simulink model "Udan_SOC"  (R2017b)
settings: Solver=FixedStepAuto  StartTime=0.0  StopTime=1000  FixedStep=0.1  RelTol=1e-3
values from neighbouring files (symbols this model uses):
  DenominatorOfIntegratorFactor = 100.0    [SOC_Stateflow.sldd]
  SOC_CalcSohLKT = 1.0    [SOC_Stateflow.sldd]
  SOC_CalcSOHTempLimit = 70.0    [SOC_Stateflow.sldd]
  SOC_CapPerCycle = 100.0    [SOC_Stateflow.sldd]
  SOC_CapTemp_HLimit = 200.0    [SOC_Stateflow.sldd]
  SOC_CapTemp_LLimit = 0.0    [SOC_Stateflow.sldd]
  Soc_ConfigInfo = 0    [SOC_Stateflow.sldd]
  SOC_DchgEndCalib = 0.0    [SOC_Stateflow.sldd]
  SOC_DiffVoltMin = 10.0    [SOC_Stateflow.sldd]
  SOC_DSOCJumpMax = 500.0    [SOC_Stateflow.sldd]
  SOC_EfficientHighLimit = 250.0    [SOC_Stateflow.sldd]
  SOC_EfficientLowLimit = 40.0    [SOC_Stateflow.sldd]
  SOC_EmptyAus = 0.0    [SOC_Stateflow.sldd]
  SOC_EnableOcv = 1.0    [SOC_Stateflow.sldd]
  SOC_END_CALIB_STATE : value not decoded    [SOC_Stateflow.sldd]
  SOC_HighRealSoc = 95.0    [SOC_Stateflow.sldd]
  SOC_LKTSohCycles = 0.0 1.0 10.0 20.0 30.0 40.0 50.0 60.0 70.0 80.0 90.0 100.0 110.0 120.0 130.0 140.0 150.0 160.0 170.0 180.0 190.0 200.0 210.0 220.0 230.0 240.0 250.0 260.0 270.0 280.0 290.0 300.0 310.0 320.0 330.0 340.0 350.0 360.0 370.0 380.0 390.0 400.0 410.0 420.0 430.0 440.0 450.0 460.0 470.0 480.0 490.0 500.0 510.0 520.0 530.0 540.0 550.0 560.0 570.0 580.0 590.0 600.0 610.0 620.0 630.0 640.0 650.0 660.0 670.0    [SOC_Stateflow.sldd]
  SOC_LKTSohTable = 1000.0 991.0 989.0 992.0 993.0 995.0 994.0 993.0 1000.0 997.0 1002.0 1000.0 992.0 1000.0 989.0 992.0 989.0 994.0 989.0 993.0 994.0 994.0 994.0 993.0 991.0 991.0 992.0 993.0 991.0 985.0 985.0 985.0 979.0 975.0 978.0 984.0 982.0 974.0 975.0 972.0 972.0 975.0 977.0 977.0 974.0 971.0 973.0 971.0 966.0 968.0 965.0 959.0 957.0 956.0 957.0 954.0 955.0 951.0 954.0 951.0 942.0 942.0 940.0 942.0 947.0 949.0    [SOC_Stateflow.sldd]
  SOC_LowRealSoc = 5.0    [SOC_Stateflow.sldd]
  SOC_NominalCap_AmS = 576000000.0    [SOC_Stateflow.sldd]
  SOC_NominalVol = 4000.0    [SOC_Stateflow.sldd]
  SOC_OCVTemp_HLimit = 106.0    [SOC_Stateflow.sldd]
  SOC_OCVTemp_LLimit = 29.0    [SOC_Stateflow.sldd]
  SOC_ShortCalibDSoc = 1.0    [SOC_Stateflow.sldd]
  SOC_SOCResolution = 10000.0    [SOC_Stateflow.sldd]
  SOC_SohCalcCapPercent = 8.0    [SOC_Stateflow.sldd]
  SOC_SohCalcHighLimit = 60.0    [SOC_Stateflow.sldd]
  SOC_SohCalcLowLimit = 10.0    [SOC_Stateflow.sldd]
  SOC_SohCalcMidLimit = 30.0    [SOC_Stateflow.sldd]
  SOC_SOHResolution = 1000.0    [SOC_Stateflow.sldd]
  SOC_State = <binary blob, 1163 chars, not shown>    [SOC_Stateflow.sldd]
  SOC_TempCap_CapBuffer : value not decoded    [SOC_Stateflow.sldd]
  SOC_TempCap_TempBuffer : value not decoded    [SOC_Stateflow.sldd]
  SocOcvCalib_ConfigInfo = 0.0    [SOC_Stateflow.sldd]
  SocOcvCalib_SocBuffer1 : value not decoded    [SOC_Stateflow.sldd]
  SocOcvCalib_TempBuffer : value not decoded    [SOC_Stateflow.sldd]
  SocOcvCalib_VoltageBuffer1 = 3300.0 3303.0 3305.0 3307.0 3310.0 3311.0 3313.0 3314.0 3316.0 3317.0 3319.0 3320.0 3322.0 3323.0 3325.0 3322.0 3323.0 3325.0 3310.0 3313.0 3315.0 3317.0 3320.0 3321.0 3323.0 3324.0 3326.0 3327.0 3329.0 3330.0 3332.0 3333.0 3335.0 3332.0 3333.0 3335.0 3320.0 3323.0 3325.0 3327.0 3330.0 3331.0 3333.0 3334.0 3336.0 3337.0 3339.0 3340.0 3342.0 3343.0 3345.0 3342.0 3343.0 3345.0 3330.0 3333.0 3335.0 3    [SOC_Stateflow.sldd]
  SOHCalibCycle = 10.0    [SOC_Stateflow.sldd]
undefined symbols (not defined in the file or in its folder): DatetimeM_GetReturnType, ParameterM_EeepParaIndexType, Soc_CumuLativeTypeType, SOC_EgthTempChgValue, Soc_EnergyBuffer, SOC_FithTempChgValue, SOC_FstSlowTempChgValue, SOC_FstTempChgValue, SOC_FthTempChgValue, SOC_MaxCap_AmS, SOC_SethTempChgValue, SOC_SixTempChgValue, SOC_SndSlowTempChgValue, SOC_SndTempChgValue, SOC_TrdSlowTempChgValue, SOC_TrdTempChgValue, SocDiagCalib_NoCalibReasonType
libraries: simulink x138, hdlsllib x24, dspindex x4
(part 4 of 10)

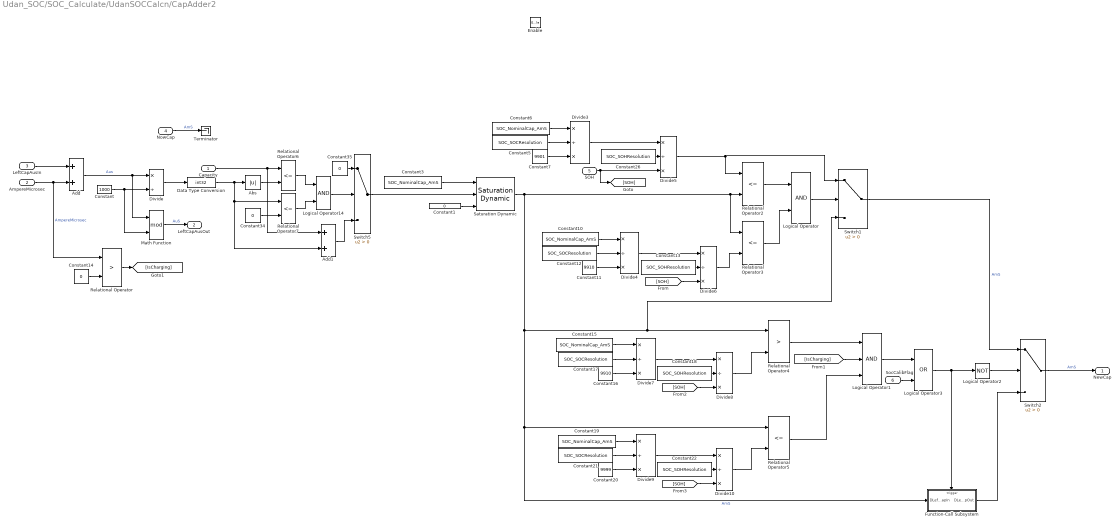
== system Udan_SOC/SOC_Calculate/UdanSOCCalcn/CapAdder2 ==
  Capacity : Inport
  AmpereMicrosec : Inport  Port=2
  LeftCapAusIn : Inport  Port=3
  NowCap : Inport  Port=4
  SOH : Inport  Port=5
  SocCalibFlag : Inport  Port=6  OutDataTypeStr=uint8  PortDimensions=[1]
  Enable : EnablePort
  Abs : Abs
  Add : Sum  AccumDataTypeStr=int32  OutDataTypeStr=int32
  Add1 : Sum  AccumDataTypeStr=uint32  OutDataTypeStr=uint32
  Constant : Constant  Value=1000  OutDataTypeStr=int32
  Constant1 : Constant  Value=0  OutDataTypeStr=uint32
  Constant{3,6,10,15,19} (5 alike) : Constant  Value=SOC_NominalCap_AmS
  Constant11 : Constant  Value=9910  OutDataTypeStr=uint16
  Constant{5,12,17,21} (4 alike) : Constant  Value=SOC_SOCResolution  OutDataTypeStr=uint16
  Constant{13,18,22,26} (4 alike) : Constant  Value=SOC_SOHResolution  OutDataTypeStr=uint16
  Constant14 : Constant  Value=0  OutDataTypeStr=uint8
  Constant16 : Constant  Value=9910  OutDataTypeStr=uint16
  Constant20 : Constant  Value=9999  OutDataTypeStr=uint16
  Constant34 : Constant  Value=0  OutDataTypeStr=uint8
  Constant35 : Constant  Value=0  OutDataTypeStr=uint8
  Constant7 : Constant  Value=9901  OutDataTypeStr=uint16
  Data Type Conversion : DataTypeConversion  OutDataTypeStr=int32
  Divide : Product  Inputs=*/  OutDataTypeStr=int32
  Divide{3..10} (8 alike) : Product  Inputs=*/*  OutDataTypeStr=uint32
  Function-Call Subsystem : Subsystem  TreatAsAtomicUnit=on
  Logical Operator : Logic  AllPortsSameDT=off  OutDataTypeStr=boolean
  Logical Operator1 : Logic  Inputs=3  AllPortsSameDT=off  OutDataTypeStr=boolean
  Logical Operator14 : Logic  AllPortsSameDT=off  OutDataTypeStr=boolean
  Logical Operator2 : Logic  Operator=NOT  AllPortsSameDT=off  OutDataTypeStr=boolean
  Logical Operator3 : Logic  Operator=OR  AllPortsSameDT=off  OutDataTypeStr=boolean
  Math Function : Math  Operator=mod  SaturateOnIntegerOverflow=on
  Relational Operator : RelationalOperator  Operator=>  OutDataTypeStr=boolean  RndMeth=Simplest
  Relational Operator{2..3,5..7} (5 alike) : RelationalOperator  Operator=<=  OutDataTypeStr=boolean  RndMeth=Simplest
  Relational Operator4 : RelationalOperator  Operator=>  OutDataTypeStr=boolean  RndMeth=Simplest
  Saturation Dynamic : simulink/Discontinuities/Saturation Dynamic  OutMin=[]  OutMax=[]  OutDataTypeStr=uint32  OutputDataTypeScalingMode=uint32  OutDataType=fixdt(1, 16)  OutScaling=2^-10  DoSatur=on
  Switch1 : Switch  Criteria=u2 > Threshold
  Switch2 : Switch  Criteria=u2 > Threshold
  Switch5 : Switch  Criteria=u2 > Threshold  OutDataTypeStr=uint32
  Terminator : Terminator
  NewCap : Outport
  LeftCapAusOut : Outport  Port=2
  wires:
  Add/1 -> Divide/1, Math Function/1  "Aus"
  Switch2/1 -> NewCap/1  "AmS"
  AmpereMicrosec/1 -> Relational Operator/1, Add/2  "AmpereMicrosec"
  Constant3/1 -> Saturation Dynamic/1
  Math Function/1 -> LeftCapAusOut/1  "AuS"
  Divide/1 -> Data Type Conversion/1
  Constant/1 -> Divide/2, Math Function/2
  LeftCapAusIn/1 -> Add/1
  Constant1/1 -> Saturation Dynamic/3
  Switch5/1 -> Saturation Dynamic/2
  Constant11/1 -> Divide4/3
  Relational Operator3/1 -> Logical Operator/2
  Divide6/1 -> Relational Operator3/2
  Logical Operator/1 -> Switch1/2
  Constant12/1 -> Divide4/2
  Constant5/1 -> Divide3/2
  Constant7/1 -> Divide3/3
  Relational Operator2/1 -> Logical Operator/1
  Saturation Dynamic/1 -> Relational Operator5/1, Function-Call Subsystem/1(DLeftCapIn), Switch1/3, Relational Operator4/1, Relational Operator3/1, Relational Operator2/2  "AmS"
  Divide5/1 -> Switch1/1, Relational Operator2/1
  Constant26/1 -> Divide5/2
  SOH/1 -> [SOH], Divide5/3
  Divide3/1 -> Divide5/1
  Constant13/1 -> Divide6/2
  Divide4/1 -> Divide6/1
  [SOH] -> Divide6/3
  Constant14/1 -> Relational Operator/2
  Relational Operator/1 -> [IsCharging]
  Divide7/1 -> Divide8/1
  Constant16/1 -> Divide7/3
  [SOH] -> Divide8/3
  Constant17/1 -> Divide7/2
  Constant18/1 -> Divide8/2
  Divide8/1 -> Relational Operator4/2
  Relational Operator4/1 -> Logical Operator1/1
  [IsCharging] -> Logical Operator1/2
  Logical Operator3/1 -> Logical Operator2/1, Function-Call Subsystem/Trigger
  Logical Operator2/1 -> Switch2/2
  Switch1/1 -> Switch2/1  "AmS"
  Function-Call Subsystem/1(DLeftCapOut) -> Switch2/3
  SocCalibFlag/1 -> Logical Operator3/2
  Logical Operator1/1 -> Logical Operator3/1
  Constant21/1 -> Divide9/2
  Divide10/1 -> Relational Operator5/2
  Constant20/1 -> Divide9/3
  [SOH] -> Divide10/3
  Constant22/1 -> Divide10/2
  Divide9/1 -> Divide10/1
  Relational Operator5/1 -> Logical Operator1/3
  Constant6/1 -> Divide3/1
  Constant10/1 -> Divide4/1
  Constant15/1 -> Divide7/1
  Constant19/1 -> Divide9/1
  NowCap/1 -> Terminator/1  "AmS"
  Logical Operator14/1 -> Switch5/2
  Relational Operator7/1 -> Logical Operator14/2
  Relational Operator6/1 -> Logical Operator14/1
  Constant35/1 -> Switch5/1
  Add1/1 -> Switch5/3
  Abs/1 -> Relational Operator6/2
  Capacity/1 -> Add1/1, Relational Operator6/1
  Constant34/1 -> Relational Operator7/2
  Data Type Conversion/1 -> Abs/1, Relational Operator7/1, Add1/2

== system Udan_SOC/SOC_Calculate/UdanSOCCalcn/ClearLeftCapWOCalib ==
  Trigger : TriggerPort  TriggerType=either  VariantControl=Variant  PortDimensions=1
  Constant2 : Constant  Value=0  OutDataTypeStr=uint32
  DchgPower2 : simulink/Sources/Enumerated Constant  OutDataTypeStr=Enum: ParameterM_EeepParaIndexType  Value=ParameterM_EeepParaIndexType.PARAMETERM_EEEP_LEFTCAP_WOCALIB_H_INDEX  SampleTime=inf
      settings: SourceProductName=Simulink
  DchgPower4 : simulink/Sources/Enumerated Constant  OutDataTypeStr=Enum: ParameterM_EeepParaIndexType  Value=ParameterM_EeepParaIndexType.PARAMETERM_EEEP_LEFTCAP_WOCALIB_L_INDEX  SampleTime=inf
      settings: SourceProductName=Simulink
  Subsystem : Subsystem  mask(EeepWrite_uint32){}
      mask help: EeepWrite_uint32
  wires:
  Constant2/1 -> Subsystem/1(data)
  DchgPower4/1 -> Subsystem/3(LowIndex)
  DchgPower2/1 -> Subsystem/2(HighIndex)

== system Udan_SOC/SOC_Calculate/UdanSOCCalcn/ClearLeftCapWOCalib2 ==
  Enable : EnablePort
  Constant : Constant  OutDataTypeStr=boolean
  Constant2 : Constant  Value=0  OutDataTypeStr=uint32
  Data Store Write : DataStoreWrite  DataStoreName=ChgClearWOCalibFlag
  DchgPower2 : simulink/Sources/Enumerated Constant  OutDataTypeStr=Enum: ParameterM_EeepParaIndexType  Value=ParameterM_EeepParaIndexType.PARAMETERM_EEEP_LEFTCAP_WOCALIB_H_INDEX  SampleTime=inf
      settings: SourceProductName=Simulink
  DchgPower4 : simulink/Sources/Enumerated Constant  OutDataTypeStr=Enum: ParameterM_EeepParaIndexType  Value=ParameterM_EeepParaIndexType.PARAMETERM_EEEP_LEFTCAP_WOCALIB_L_INDEX  SampleTime=inf
      settings: SourceProductName=Simulink
  Subsystem : Subsystem  mask(EeepWrite_uint32){}
      mask help: EeepWrite_uint32
  wires:
  DchgPower2/1 -> Subsystem/2(HighIndex)
  Constant2/1 -> Subsystem/1(data)
  DchgPower4/1 -> Subsystem/3(LowIndex)
  Constant/1 -> Data Store Write/1

== system Udan_SOC/SOC_Calculate/UdanSOCCalcn/ClearSOHCalcFlag ==
  Enable : EnablePort
  Constant1 : Constant  Value=65535  OutDataTypeStr=uint16
  DchgPower1 : simulink/Sources/Enumerated Constant  OutDataTypeStr=Enum: ParameterM_EeepParaIndexType  Value=ParameterM_EeepParaIndexType.PARAMETERM_EEEP_SOH_Full_INDEX  SampleTime=inf
      settings: SourceProductName=Simulink
  S-Function1 : S-Function  FunctionName=sfn_NVMWrite  SFunctionDeploymentMode=off  EnableBusSupport=off
  Terminator : Terminator
  wires:
  DchgPower1/1 -> S-Function1/1
  S-Function1/1 -> Terminator/1
  Constant1/1 -> S-Function1/2

== system Udan_SOC/SOC_Calculate/UdanSOCCalcn/Enabled Subsystem ==
  RtcTimeIn : Inport
  Enable : EnablePort
  Constant : Constant  OutDataTypeStr=boolean
  Data Store Write : DataStoreWrite  DataStoreName=LargeCurrentFlag
  RtcTimeOut : Outport
  wires:
  RtcTimeIn/1 -> RtcTimeOut/1
  Constant/1 -> Data Store Write/1

== system Udan_SOC/SOC_Calculate/UdanSOCCalcn/Function-Call Subsystem ==
  function : TriggerPort  TriggerType=falling  VariantControl=Variant
  Constant : Constant  Commented=on  Value=0  OutDataTypeStr=boolean
  Constant1 : Constant  Value=0  OutDataTypeStr=boolean
  Constant2 : Constant  Value=0  OutDataTypeStr=uint32
  Data Store Write : DataStoreWrite  Commented=on  DataStoreName=FullFnshFlag
  Data Store Write1 : DataStoreWrite  DataStoreName=ChgClearWOCalibFlag
  DchgPower2 : simulink/Sources/Enumerated Constant  OutDataTypeStr=Enum: ParameterM_EeepParaIndexType  Value=ParameterM_EeepParaIndexType.PARAMETERM_EEEP_LEFTCAP_WOCALIB_H_INDEX  SampleTime=inf
      settings: SourceProductName=Simulink
  DchgPower4 : simulink/Sources/Enumerated Constant  OutDataTypeStr=Enum: ParameterM_EeepParaIndexType  Value=ParameterM_EeepParaIndexType.PARAMETERM_EEEP_LEFTCAP_WOCALIB_L_INDEX  SampleTime=inf
      settings: SourceProductName=Simulink
  Subsystem : Subsystem  mask(EeepWrite_uint32){}
      mask help: EeepWrite_uint32
  wires:
  Constant/1 -> Data Store Write/1
  DchgPower4/1 -> Subsystem/3(LowIndex)
  Constant2/1 -> Subsystem/1(data)
  DchgPower2/1 -> Subsystem/2(HighIndex)
  Constant1/1 -> Data Store Write1/1

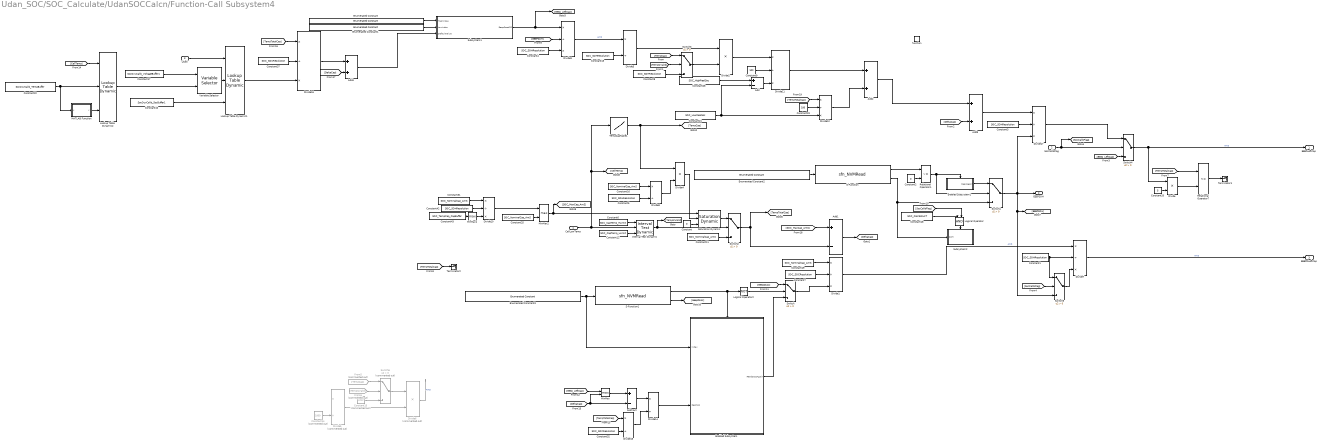
== system Udan_SOC/SOC_Calculate/UdanSOCCalcn/Function-Call Subsystem4 ==
  CellLowTemp : Inport
  SocCalibFlag : Inport  Port=2  OutDataTypeStr=uint8  PortDimensions=[1]
  UCell : Inport  Port=3
  function : TriggerPort  TriggerType=function-call  VariantControl=Variant
  Add : Sum  Inputs=+-  AccumDataTypeStr=uint8  OutDataTypeStr=uint8
  Add1 : Sum  Inputs=+-  OutDataTypeStr=int32
  Add2 : Sum  OutDataTypeStr=uint32
  Add3 : Sum  OutDataTypeStr=uint32
  Add4 : Sum
  Constant : Constant  Value=0  OutDataTypeStr=uint8
  Constant{1,3..5,8,13,42} (7 alike) : Constant  Value=SOC_SOHResolution  OutDataTypeStr=uint16
  Constant10 : Constant  Value=SocOcvCalib_SocBuffer1
  Constant{11,16,19,25,31} (5 alike) : Constant  Value=SOC_NominalCap_AmS
  Constant12 : Constant  Value=SOC_CapTemp_LLimit  OutDataTypeStr=uint8
  Constant14 : Constant  Commented=on  Value=1000  OutDataTypeStr=uint16
  Constant15 : Constant  Commented=on  Value=1000  OutDataTypeStr=uint16
  Constant17 : Constant  Value=SocOcvCalib_VoltageBuffer1
  Constant18 : Constant  Value=SOC_CalcSohLKT
  Constant2 : Constant  Value=0  OutDataTypeStr=uint8
  Constant20 : Constant  Value=5  OutDataTypeStr=uint8
  Constant21 : Constant  Value=SOC_LowRealSoc
  Constant22 : Constant  Value=SocOcvCalib_TempBuffer  OutDataTypeStr=uint8
  Constant23 : Constant  Value=100  OutDataTypeStr=uint8
  Constant28 : Constant  Value=SOC_HighRealSoc
  Constant32 : Constant  Value=SOC_SOCResolution  OutDataTypeStr=uint16
  Constant37 : Constant  Value=SOC_SOCResolution  OutDataTypeStr=uint16
  Constant43 : Constant  Value=SOC_TempCap_CapBuffer
  Constant6 : Constant  Value=SOC_CapTemp_HLimit  OutDataTypeStr=uint8
  Constant7 : Constant  Value=SOC_SOCResolution  OutDataTypeStr=uint16
  Constant9 : Constant  Value=100  OutDataTypeStr=uint8
  Divide : Product  Inputs=**  OutDataTypeStr=uint32
  Divide{1,7,9..11,16..17} (7 alike) : Product  Inputs=*/*  OutDataTypeStr=uint32
  Divide12 : Product  Inputs=*/*
  Divide14 : Product  Inputs=*/
  Divide15 : Product  Inputs=*/
  Divide2 : Product  Inputs=**  OutDataTypeStr=uint32
  Divide3 : Product  Inputs=*/  OutDataTypeStr=uint32
  Divide4 : Product  Inputs=**  OutDataTypeStr=uint32
  Divide5 : Product  Commented=on  Inputs=*/  OutDataTypeStr=uint32
  Divide6 : Product  Commented=on  Inputs=**  OutDataTypeStr=uint32
  Divide8 : Product  Inputs=*/  OutDataTypeStr=uint32
  Enabled Subsystem : Subsystem  TreatAsAtomicUnit=on
  Enabled Subsystem1 : Subsystem  TreatAsAtomicUnit=on
  Enumerated Constant : simulink/Sources/Enumerated Constant  OutDataTypeStr=Enum: ParameterM_EeepParaIndexType  Value=ParameterM_EeepParaIndexType.PARAMETERM_EEEP_LEFTCAP_H_INDEX  SampleTime=inf
      settings: SourceProductName=Simulink
  Enumerated Constant1 : simulink/Sources/Enumerated Constant  OutDataTypeStr=Enum: ParameterM_EeepParaIndexType  Value=ParameterM_EeepParaIndexType.PARAMETERM_EEEP_LEFTCAP_L_INDEX  SampleTime=inf
      settings: SourceProductName=Simulink
  Enumerated Constant2 : simulink/Sources/Enumerated Constant  OutDataTypeStr=Enum: ParameterM_EeepParaIndexType  Value=ParameterM_EeepParaIndexType.PARAMETERM_EEEP_SOH_INDEX  SampleTime=inf
      settings: SourceProductName=Simulink
  Enumerated Constant3 : simulink/Sources/Enumerated Constant  OutDataTypeStr=Enum: ParameterM_EeepParaIndexType  Value=ParameterM_EeepParaIndexType.PARAMETERM_EEEP_MODEL_DSOC_INDEX  SampleTime=inf
      settings: SourceProductName=Simulink
  From5 : From  Commented=on  GotoTag=TempCap
  From6 : From  Commented=on  GotoTag=TempIsValid
  Interval Test Dynamic : simulink/Logic and Bit Operations/Interval Test Dynamic  IntervalClosedRight=off  IntervalClosedLeft=off  OutDataTypeStr=boolean
      settings: SourceProductName=Simulink  SourceProductBaseCode=SL
  Logical Operator : Logic  AllPortsSameDT=off  OutDataTypeStr=boolean
  Logical Operator2 : Logic  Operator=NOT  AllPortsSameDT=off  OutDataTypeStr=boolean
  Lookup Table Dynamic1 : simulink/Lookup Tables/Lookup Table Dynamic  LookUpMeth=Interpolation-Use End Values  OutDataType=fixdt('uint16')  OutScaling=[]  OutputDataTypeScalingMode=Specify via dialog  OutDataTypeStr=uint16  DoSatur=on
      settings: SourceProductName=Simulink
  Lookup Table Dynamic2 : simulink/Lookup Tables/Lookup Table Dynamic  LookUpMeth=Use Input Nearest  OutDataType=fixdt('uint8')  OutScaling=[]  OutputDataTypeScalingMode=Specify via dialog  OutDataTypeStr=uint8  DoSatur=on
      settings: SourceProductName=Simulink
  MATLAB Function : MATLAB Function  TreatAsAtomicUnit=on
  MinMax : MinMax  Function=max  Inputs=2
  MinMax1 : MinMax  Function=max
  MinMax2 : MinMax  Function=max  Inputs=2
  Relational Operator1 : RelationalOperator  Operator=~=  OutDataTypeStr=boolean  RndMeth=Simplest
  Relational Operator7 : RelationalOperator  Operator=<=  OutDataTypeStr=boolean  RndMeth=Simplest
  S-Function : S-Function  FunctionName=sfn_NVMRead  SFunctionDeploymentMode=off  EnableBusSupport=off
  S-Function1 : S-Function  FunctionName=sfn_NVMRead  SFunctionDeploymentMode=off  EnableBusSupport=off
  Saturation Dynamic : simulink/Discontinuities/Saturation Dynamic  OutMin=[]  OutMax=[]  OutDataTypeStr=Inherit: Same as second input  OutDataType=fixdt(1, 16)  OutScaling=2^-10  DoSatur=off
  Subsystem1 : Subsystem  mask(ReadEeep_uint32){}
  Subsystem2 : Subsystem
  Subtract : Sum  Inputs=+-  AccumDataTypeStr=int32  OutDataTypeStr=int32
  Switch{,1..3,5} (5 alike) : Switch  Criteria=u2 > Threshold
  Switch4 : Switch  Criteria=u2 > Threshold  OutDataTypeStr=uint32
  Switch6 : Switch  Commented=on  Criteria=u2 > Threshold
  TempCapTable1 : Lookup_n-D  NumberOfTableDimensions=1  BreakpointsForDimension1=SOC_TempCap_TempBuffer  Table=SOC_TempCap_CapBuffer  ExtrapMethod=Clip  InternalRulePriority=Speed  OutDataTypeStr=uint16  RndMeth=Simplest  InputSameDT=on
  Terminator1 : Terminator
  Terminator2 : Terminator
  Variable Selector : dspindex/Variable Selector  NumInputs=1  rowsOrCols=Rows  IdxMode=Variable  Elements=[1 3]  ZerOneIdxMode=One-based  errmode=Clip Index  FillMode=on  FillValues=0
  EEEPLeftCap : Outport
  EEEPSOH : Outport  Port=2
  EEEPDLeftCap : Outport  Port=3
  wires:
  S-Function/2 -> Subsystem2/1(SOH), Switch1/3
  Constant2/1 -> Relational Operator1/2
  S-Function/1 -> Relational Operator1/1
  Enumerated Constant2/1 -> S-Function/1
  Add4/1 -> Subsystem1/3(DefaultValue)
  Enumerated Constant1/1 -> Subsystem1/2(LowIndex)
  Enumerated Constant/1 -> Subsystem1/1(HighIndex)
  Switch1/1 -> Divide17/3, Switch5/3, [EEEPSOH], EEEPSOH/1
  Switch4/1 -> Divide/1, EEEPLeftCap/1  "AmS"
  [SOC_MaxCap_AmS] -> Add1/1
  Switch2/1 -> Add1/2, [TempTotalCap]
  Enumerated Constant3/1 -> Enabled Subsystem/1(Index), S-Function1/1
  S-Function1/2 -> [EeepDsoc]
  Divide4/1 -> Saturation Dynamic/2
  Constant6/1 -> Interval Test Dynamic/1
  Interval Test Dynamic/1 -> [TempIsValid], Switch2/2
  Divide8/1 -> Divide4/2
  Constant12/1 -> Interval Test Dynamic/3
  CellLowTemp/1 -> [CellTemp], TempCapTable1/1, Interval Test Dynamic/2
  Constant7/1 -> Divide1/2
  S-Function1/1 -> Enabled Subsystem/Enable, Logical Operator2/1
  Add1/1 -> [DeltaCap]
  Switch3/1 -> Divide2/2
  [TempCap] -> Switch3/1
  [TempIsValid] -> Switch3/2
  Constant8/1 -> Switch3/3
  Add2/1 -> Add3/1
  [DeltaCap] -> Add3/2
  SocCalibFlag/1 -> [SocCalibFlag], Switch4/2
  Divide17/1 -> Switch4/1
  [Eeep_LeftCap] -> Switch4/3
  Divide3/1 -> Divide2/1
  Constant13/1 -> Divide3/2
  Constant14/1 -> Divide5/2
  Constant15/1 -> Switch6/3
  Switch6/1 -> Divide6/1
  From5/1 -> Switch6/1
  From6/1 -> Switch6/2
  Divide5/1 -> Divide6/2
  Divide6/1 -> ?  "AmS"
  Divide1/1 -> Divide7/1  "AmS"
  Constant1/1 -> Switch5/1, Divide7/2
  [SocCalibFlag] -> Switch5/2
  Switch5/1 -> Divide7/3
  Constant5/1 -> Divide8/2
  TempCapTable1/1 -> Divide4/1, [TempCap]
  Divide/1 -> Relational Operator7/2
  Constant20/1 -> Divide/2
  [TempTotalCap] -> Relational Operator7/1
  Relational Operator7/1 -> Terminator1/1
  Divide7/1 -> EEEPDLeftCap/1  "AmS"
  Constant19/1 -> Divide1/1
  [TempTotalCap] -> Terminator2/1
  [Eeep_LeftCap] -> MinMax/1
  [DeltaCap] -> MinMax/2, Subtract/2
  Subtract/1 -> Divide14/1
  [TempTotalCap] -> Divide15/1
  Constant32/1 -> Divide15/2
  Divide15/1 -> Divide14/2
  MinMax/1 -> Subtract/1
  Divide14/1 -> Enabled Subsystem/2(RealSoc)
  Constant22/1 -> MATLAB Function/1(u), Lookup Table Dynamic2/2
  Variable Selector/1 -> Lookup Table Dynamic1/2
  Lookup Table Dynamic1/1 -> Divide16/3
  MATLAB Function/1(y) -> Lookup Table Dynamic2/3
  Lookup Table Dynamic2/1 -> Variable Selector/2
  UCell/1 -> Lookup Table Dynamic1/1
  [CellTemp] -> Lookup Table Dynamic2/1
  [TempTotalCap] -> Divide16/1
  Constant37/1 -> Divide16/2
  Divide16/1 -> Add4/1
  [DeltaCap] -> Add4/2
  Switch/1 -> Divide1/3
  Enabled Subsystem/1(ReadDsocAgain) -> Switch/3
  Logical Operator2/1 -> Switch/2
  [EeepDsoc] -> Switch/1
  Relational Operator1/1 -> Switch1/2, Enabled Subsystem1/Enable
  Enabled Subsystem1/1(ReadAgain) -> Switch1/1
  Constant3/1 -> Divide17/2
  Add3/1 -> Divide17/1
  Subsystem1/1(EeepRead32) -> [Eeep_LeftCap], Divide9/1
  Constant4/1 -> Divide9/3
  [EEEPSOH] -> Divide9/2
  [SocCalibFlag] -> Logical Operator/2
  Saturation Dynamic/1 -> Switch2/1
  MinMax2/1 -> [SOC_MaxCap_AmS], Saturation Dynamic/1
  Constant/1 -> Saturation Dynamic/3
  Logical Operator/1 -> Subsystem2/Enable
  Constant10/1 -> Lookup Table Dynamic1/3
  Constant17/1 -> Variable Selector/1
  Divide9/1 -> Divide3/1  "AmS"
  Divide2/1 -> Divide11/1
  Constant9/1 -> Divide11/2
  Constant21/1 -> Add/2, Divide12/3
  Add/1 -> Divide11/3
  [TempTotalCap] -> Divide12/1
  Constant23/1 -> Divide12/2
  Divide11/1 -> Add2/1
  Divide12/1 -> Add2/2
  Constant11/1 -> Switch2/3
  Constant16/1 -> Divide8/1
  Constant28/1 -> Add/1
  Constant18/1 -> Logical Operator/1
  Constant42/1 -> Divide10/2
  Constant43/1 -> MinMax1/1
  MinMax1/1 -> Divide10/3
  Divide10/1 -> MinMax2/1
  Constant25/1 -> MinMax2/2
  Constant31/1 -> Divide10/1

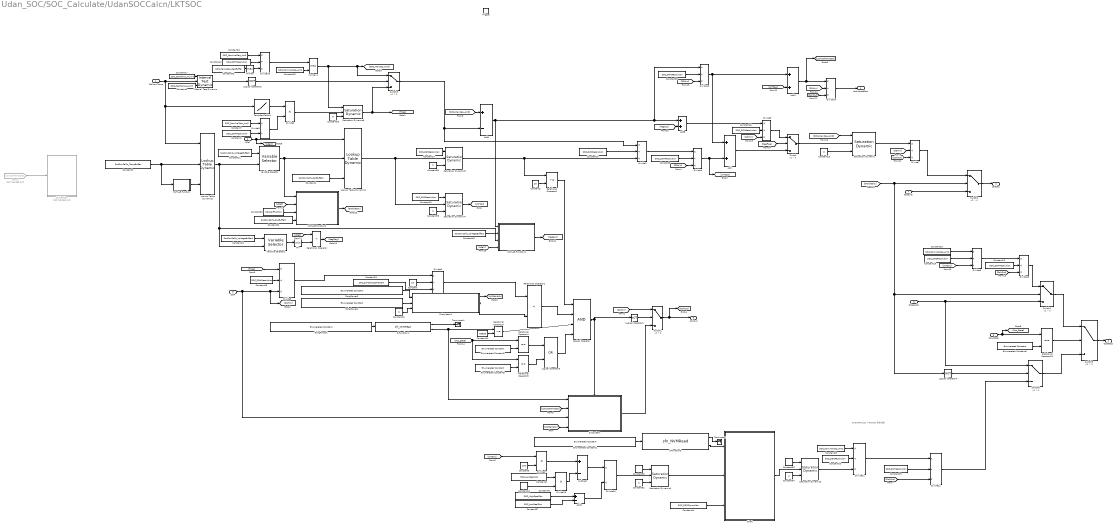
== system Udan_SOC/SOC_Calculate/UdanSOCCalcn/LKTSOC ==
  note: DK300PackSoc与RealSoc策略调整
  CellLowTemp : Inport
  UCell : Inport  Port=2
  SOH : Inport  Port=3
  Capacity : Inport  Port=4
  DCapacity : Inport  Port=5
  Soc_State : Inport  Port=6
  Trigger : TriggerPort  TriggerType=function-call  VariantControl=Variant  PortDimensions=1
  Add : Sum  AccumDataTypeStr=uint32  OutDataTypeStr=uint32
  Add1 : Sum  Inputs=+-  OutDataTypeStr=int32
  Add2 : Sum  Inputs=+-  AccumDataTypeStr=uint8  OutDataTypeStr=uint8
  Add4 : Sum  AccumDataTypeStr=int32  OutDataTypeStr=int32
  Add5 : Sum  AccumDataTypeStr=int32  OutDataTypeStr=int32
  CalcLeftCap : Subsystem  Commented=on
  Chart : Stateflow chart  TreatAsAtomicUnit=on
  Constant : Constant  Value=10  OutDataTypeStr=uint8
  Constant{1,8,13,15,29,38,42,46} (8 alike) : Constant  Value=SOC_SOHResolution  OutDataTypeStr=uint16
  Constant{10,19,26..27,40} (5 alike) : Constant  Value=SOC_SOCResolution  OutDataTypeStr=uint16
  Constant11 : Constant  Value=SocOcvCalib_VoltageBuffer1
  Constant12 : Constant  Value=10000  OutDataTypeStr=uint16
  Constant14 : Constant  Value=65535  OutDataTypeStr=uint16
  Constant16 : Constant  Value=0  OutDataTypeStr=uint32
  Constant17 : Constant  Value=SOC_CapTemp_HLimit  OutDataTypeStr=uint8
  Constant18 : Constant  Value=0  OutDataTypeStr=uint8
  Constant2 : Constant  Value=20  OutDataTypeStr=uint16
  Constant{7,20,25,28,31} (5 alike) : Constant  Value=SOC_NominalCap_AmS
  Constant21 : Constant  Value=SocOcvCalib_VoltageBuffer1
  Constant22 : Constant  Value=SocOcvCalib_SocBuffer1
  Constant23 : Constant  Value=0  OutDataTypeStr=uint16
  Constant24 : Constant  Value=SOC_SohCalcCapPercent  OutDataTypeStr=uint8
  Constant3 : Constant  Value=SocOcvCalib_TempBuffer  OutDataTypeStr=uint8
  Constant30 : Constant  Value=SOC_DiffVoltMin
  Constant{32,34,36,39} (4 alike) : Constant  Value=2  OutDataTypeStr=uint16
  Constant33 : Constant  Value=10001  OutDataTypeStr=uint16
  Constant35 : Constant  Value=10001  OutDataTypeStr=uint16
  Constant37 : Constant  Value=SOC_LowRealSoc
  Constant4 : Constant  Value=SocOcvCalib_SocBuffer1
  Constant41 : Constant  Value=SOC_HighRealSoc
  Constant43 : Constant  Value=SOC_TempCap_CapBuffer
  Constant44 : Constant  Value=SOC_DSOCJumpMax
  Constant45 : Constant  Value=SocOcvCalib_VoltageBuffer1
  Constant5 : Constant  Value=100  OutDataTypeStr=uint8
  Constant6 : Constant  Value=SOC_LowRealSoc
  Constant9 : Constant  Value=SOC_CapTemp_LLimit  OutDataTypeStr=uint8
  DchgPower1 : simulink/Sources/Enumerated Constant  OutDataTypeStr=Enum: ParameterM_EeepParaIndexType  Value=ParameterM_EeepParaIndexType.PARAMETERM_EEEP_SOH_Full_INDEX  SampleTime=inf
      settings: SourceProductName=Simulink
  DchgPower2 : simulink/Sources/Enumerated Constant  OutDataTypeStr=Enum: ParameterM_EeepParaIndexType  Value=ParameterM_EeepParaIndexType.PARAMETERM_EEEP_LEFTCAP_WOCALIB_H_INDEX  SampleTime=inf
      settings: SourceProductName=Simulink
  DchgPower4 : simulink/Sources/Enumerated Constant  OutDataTypeStr=Enum: ParameterM_EeepParaIndexType  Value=ParameterM_EeepParaIndexType.PARAMETERM_EEEP_LEFTCAP_WOCALIB_L_INDEX  SampleTime=inf
      settings: SourceProductName=Simulink
  Divide{1,4..9,11..16} (13 alike) : Product  Inputs=*/*  OutDataTypeStr=uint32
  Divide17 : Product  Inputs=**  OutDataTypeStr=uint32
  Divide18 : Product  Inputs=**  OutDataTypeStr=uint32
  Divide19 : Product  Inputs=*/  OutDataTypeStr=int32
  Divide2 : Product  Inputs=**  OutDataTypeStr=uint32
  Divide3 : Product  Inputs=*/  OutDataTypeStr=uint32
  Enumerated Constant1 : simulink/Sources/Enumerated Constant  OutDataTypeStr=Enum: ParameterM_EeepParaIndexType  Value=ParameterM_EeepParaIndexType.PARAMETERM_EEEP_MODEL_DSOC_INDEX  SampleTime=inf
      settings: SourceProductName=Simulink
  Enumerated Constant2 : simulink/Sources/Enumerated Constant  OutDataTypeStr=Enum: SOC_State  Value=SOC_State.SOC_STATE_OCV_LONG  SampleTime=inf
      settings: SourceProductName=Simulink
  Enumerated Constant3 : simulink/Sources/Enumerated Constant  OutDataTypeStr=Enum: SOC_State  Value=SOC_State.SOC_STATE_OCV  SampleTime=inf
      settings: SourceProductName=Simulink
  Enumerated Constant6 : simulink/Sources/Enumerated Constant  OutDataTypeStr=Enum: SOC_State  Value=SOC_State.SOC_STATE_OCV_LONG  SampleTime=inf
      settings: SourceProductName=Simulink
  From1 : From  Commented=on  GotoTag=LookUpTempCap
  Interval Test Dynamic : simulink/Logic and Bit Operations/Interval Test Dynamic  IntervalClosedRight=off  IntervalClosedLeft=off  OutDataTypeStr=boolean
      settings: SourceProductName=Simulink  SourceProductBaseCode=SL
  Logical Operator : Logic  Inputs=4  AllPortsSameDT=off  OutDataTypeStr=boolean
  Logical Operator1 : Logic  Operator=NOT  AllPortsSameDT=off  OutDataTypeStr=boolean
  Logical Operator2 : Logic  Operator=NOT  AllPortsSameDT=off  OutDataTypeStr=boolean
  Logical Operator3 : Logic  Operator=OR  AllPortsSameDT=off  OutDataTypeStr=boolean
  Logical Operator4 : Logic  Operator=NOT  AllPortsSameDT=off  OutDataTypeStr=boolean
  Lookup Table Dynamic1 : simulink/Lookup Tables/Lookup Table Dynamic  LookUpMeth=Interpolation-Use End Values  OutDataType=fixdt('uint16')  OutScaling=[]  OutputDataTypeScalingMode=Specify via dialog  OutDataTypeStr=uint16  DoSatur=on
      settings: SourceProductName=Simulink
  Lookup Table Dynamic2 : simulink/Lookup Tables/Lookup Table Dynamic  LookUpMeth=Use Input Nearest  OutDataType=fixdt('uint8')  OutScaling=[]  OutputDataTypeScalingMode=Specify via dialog  OutDataTypeStr=uint8  DoSatur=on
      settings: SourceProductName=Simulink
  MATLAB Function : MATLAB Function  TreatAsAtomicUnit=on
  MATLAB Function1 : MATLAB Function  TreatAsAtomicUnit=on
  MATLAB Function2 : MATLAB Function  TreatAsAtomicUnit=on
  Min : MinMax
  MinMax : MinMax  Function=max
  MinMax1 : MinMax  Function=max  Inputs=2
  Relational Operator : RelationalOperator  Operator=<  OutDataTypeStr=boolean  RndMeth=Simplest
  Relational Operator1 : RelationalOperator  Operator=<  OutDataTypeStr=boolean  RndMeth=Simplest
  Relational Operator10 : RelationalOperator  Operator===  OutDataTypeStr=boolean  RndMeth=Simplest
  Relational Operator2 : RelationalOperator  OutDataTypeStr=boolean  RndMeth=Simplest
  Relational Operator3 : RelationalOperator  Operator=~=  OutDataTypeStr=boolean  RndMeth=Simplest
  Relational Operator4 : RelationalOperator  Operator===  OutDataTypeStr=boolean  RndMeth=Simplest
  Relational Operator5 : RelationalOperator  Operator===  OutDataTypeStr=boolean  RndMeth=Simplest
  S-Function1 : S-Function  FunctionName=sfn_NVMRead  SFunctionDeploymentMode=off  EnableBusSupport=off
  S-Function3 : S-Function  FunctionName=sfn_NVMRead  SFunctionDeploymentMode=off  EnableBusSupport=off
  Saturation Dynamic : simulink/Discontinuities/Saturation Dynamic  OutMin=[]  OutMax=[]  OutDataTypeStr=uint32  OutputDataTypeScalingMode=uint32  OutDataType=fixdt(1, 16)  OutScaling=2^-10  DoSatur=off
  Saturation Dynamic{1..5} (5 alike) : simulink/Discontinuities/Saturation Dynamic  OutMin=[]  OutMax=[]  OutDataTypeStr=Inherit: Same as second input  OutDataType=fixdt(1, 16)  OutScaling=2^-10  DoSatur=off
  Subsystem : Subsystem
  Subsystem1 : Subsystem  mask(ReadEeep_uint32){}
  Subtract : Sum  Inputs=+-  AccumDataTypeStr=int32  OutDataTypeStr=int32
  Switch : Switch  Criteria=u2 > Threshold  OutDataTypeStr=uint32
  Switch{1..6} (6 alike) : Switch  Criteria=u2 > Threshold
  TempCapTable1 : Lookup_n-D  NumberOfTableDimensions=1  BreakpointsForDimension1=SOC_TempCap_TempBuffer  Table=SOC_TempCap_CapBuffer  ExtrapMethod=Clip  InternalRulePriority=Speed  OutDataTypeStr=uint16  RndMeth=Simplest  InputSameDT=on
  Terminator : Terminator
  Terminator1 : Terminator
  Variable Selector : dspindex/Variable Selector  NumInputs=1  rowsOrCols=Rows  IdxMode=Variable  Elements=[1 3]  ZerOneIdxMode=One-based  errmode=Clip Index  FillMode=on  FillValues=0
  Variable Selector1 : dspindex/Variable Selector  NumInputs=1  rowsOrCols=Rows  IdxMode=Variable  Elements=[1 3]  ZerOneIdxMode=One-based  errmode=Clip Index  FillMode=on  FillValues=0
  LeftCap : Outport
  DLeftCap : Outport  Port=2
  SohOut : Outport  Port=3
  LookUpLeftCap : Outport  Port=4
  wires:
  UCell/1 -> [UCell], Lookup Table Dynamic1/1
  MATLAB Function/1(y) -> Lookup Table Dynamic2/3
  Constant3/1 -> MATLAB Function/1(u), Lookup Table Dynamic2/2
  Constant4/1 -> Lookup Table Dynamic1/3
  Variable Selector/1 -> MATLAB Function2/1(cellTable), Lookup Table Dynamic1/2
  Saturation Dynamic3/1 -> Relational Operator2/1, Divide1/3  "soc"
  [enableOcv] -> Switch2/2, Logical Operator4/1, Switch4/2
  Constant2/1 -> Relational Operator2/2
  Constant7/1 -> Divide3/1
  Divide3/1 -> Divide2/2
  CellLowTemp/1 -> Interval Test Dynamic/2, TempCapTable1/1, Lookup Table Dynamic2/1
  Constant1/1 -> Divide3/2
  TempCapTable1/1 -> Divide2/1
  Constant10/1 -> Divide1/2
  Divide1/1 -> Divide4/1  "当前可用剩余容量"
  Constant8/1 -> Divide4/2
  [SOC_MaxCap_AmS] -> Add1/1
  From1/1 -> CalcLeftCap/2(LookUpTempCap)
  Saturation Dynamic/1 -> Divide7/1
  Relational Operator1/1 -> Logical Operator/2
  [SOHIn] -> Switch1/1
  Constant16/1 -> Subsystem1/3(DefaultValue)
  S-Function1/2 -> Subsystem/1(SOC_LeftCap0), Relational Operator3/1
  Subsystem1/1(EeepRead32) -> [WOCalibAh], Relational Operator1/2
  S-Function1/1 -> Terminator1/1
  Logical Operator/1 -> Logical Operator1/1, Subsystem/Enable
  Constant/1 -> Divide6/2
  [TCap] -> Divide5/1
  Subsystem/1(SohOut) -> Switch1/3
  Constant14/1 -> Relational Operator3/2
  DchgPower2/1 -> Subsystem1/1(HighIndex)
  Divide5/1 -> Divide6/1
  Divide6/1 -> Relational Operator1/1
  Relational Operator3/1 -> Logical Operator/3
  DchgPower1/1 -> S-Function1/1
  Logical Operator1/1 -> Switch1/2
  Constant15/1 -> Divide5/2
  [WOCalibAh] -> Subsystem/4(WOCalibAh)
  DchgPower4/1 -> Subsystem1/2(LowIndex)
  SOH/1 -> [SOHIn], Divide5/3, Subsystem/3(SOHIn)
  Switch3/1 -> Add1/2, Divide1/1  "Qt"
  [LookUpTempCap] -> Subsystem/2(SOC_LeftCap2)
  Capacity/1 -> Switch2/3
  [SOHIn] -> Divide4/3
  Divide7/1 -> Switch2/1
  [SOHIn] -> Divide7/2
  Constant9/1 -> Interval Test Dynamic/3
  Constant17/1 -> Interval Test Dynamic/1
  Interval Test Dynamic/1 -> Logical Operator2/1
  Logical Operator2/1 -> Switch3/2
  MinMax1/1 -> Saturation Dynamic5/1, [SOC_MaxCap_AmS], Switch3/1
  Constant19/1 -> Divide8/2
  Divide15/1 -> Switch4/1
  Switch5/1 -> DLeftCap/1
  [SOC_MaxCap_AmS] -> Saturation Dynamic/1
  Constant23/1 -> Saturation Dynamic/3
  Constant24/1 -> Divide6/3
  Relational Operator2/1 -> Logical Operator/1
  S-Function3/1 -> Terminator/1
  S-Function3/2 -> Chart/1(PackSoc)
  Enumerated Constant1/1 -> S-Function3/1
  Constant28/1 -> Divide11/1
  Constant26/1 -> Divide11/2
  Divide11/1 -> Divide12/1
  Constant29/1 -> Divide12/2
  [SohOut] -> Divide12/3
  Switch4/1 -> Switch5/1
  Divide12/1 -> Switch6/3
  Enumerated Constant6/1 -> Relational Operator10/2
  Soc_State/1 -> [Soc_State], Relational Operator10/1
  Relational Operator10/1 -> Switch5/2
  Saturation Dynamic1/1 -> Chart/2(RealSoc)
  [LKTSoc] -> Divide8/3
  Constant32/1 -> Saturation Dynamic1/3
  Constant33/1 -> Saturation Dynamic1/1
  Constant34/1 -> Saturation Dynamic2/3
  Chart/1(PackSocOut) -> Saturation Dynamic2/2
  Constant35/1 -> Saturation Dynamic2/1
  Saturation Dynamic2/1 -> Divide11/3
  Switch2/1 -> LeftCap/1
  Lookup Table Dynamic1/1 -> Saturation Dynamic4/2, Saturation Dynamic3/2
  Constant36/1 -> Saturation Dynamic3/3
  Divide13/1 -> Add/1, Add4/1
  Add1/1 -> MATLAB Function1/1(DeltaCap), Add5/1, Divide13/1  "当前可用剩余容量"
  [LKTCap] -> Add4/2
  Switch1/1 -> [SohOut], SohOut/1
  Add4/1 -> Divide14/1, [LookUpTempCap]
  [SOHIn] -> Divide14/2
  Constant38/1 -> Divide13/2
  [SOHIn] -> Divide13/3
  Divide4/1 -> [LKTCap], Add/2
  Saturation Dynamic5/1 -> Switch3/3, [TCap]
  Constant13/1 -> Divide15/2
  Divide8/1 -> Divide15/1
  [SohOut] -> Divide15/3
  Divide14/1 -> LookUpLeftCap/1
  Enumerated Constant2/1 -> Relational Operator4/2
  [Soc_State] -> Relational Operator5/1, Relational Operator4/1
  Enumerated Constant3/1 -> Relational Operator5/2
  Relational Operator4/1 -> Logical Operator3/1
  Relational Operator5/1 -> Logical Operator3/2
  Logical Operator3/1 -> Logical Operator/4
  Constant39/1 -> Saturation Dynamic4/3
  Constant40/1 -> Saturation Dynamic4/1
  Saturation Dynamic4/1 -> [LKTSoc]
  MinMax/1 -> Divide16/3
  Constant31/1 -> Divide16/1
  Constant42/1 -> Divide16/2
  Constant43/1 -> MinMax/1
  Divide2/1 -> Saturation Dynamic5/2
  Constant18/1 -> Saturation Dynamic5/3
  Constant11/1 -> Variable Selector/1
  [LKTSoc] -> Divide17/1  "soc"
  Constant27/1 -> Saturation Dynamic3/1
  Constant20/1 -> Divide8/1
  Constant37/1 -> Add2/2
  Constant6/1 -> Divide18/1
  Constant12/1 -> Divide18/2
  Subtract/1 -> Divide19/1
  Divide17/1 -> Subtract/1
  Divide18/1 -> Subtract/2
  Constant41/1 -> Add2/1
  Add2/1 -> Divide19/2
  Constant5/1 -> Divide17/2
  Divide19/1 -> Saturation Dynamic1/2
  Constant44/1 -> Chart/3(DSocJumpMax)
  [UCell] -> Relational Operator/1
  MATLAB Function1/1(LKTCap) -> [NegSoc]
  Constant45/1 -> MATLAB Function1/2(VoltBuffer)
  [UCell] -> MATLAB Function1/4(vol)
  Relational Operator/1 -> [NegFlag]
  Min/1 -> Relational Operator/2
  Variable Selector1/1 -> Min/1
  Lookup Table Dynamic2/1 -> Variable Selector1/2, MATLAB Function1/3(Index), Variable Selector/2
  Constant21/1 -> Variable Selector1/1
  [NegSoc] -> Add5/2
  [SohOut] -> Divide7/3
  [SohOut] -> Divide14/3
  Add5/1 -> Divide9/1  "当前可用剩余容量"
  [SOHIn] -> Divide9/3
  Constant46/1 -> Divide9/2
  Divide9/1 -> Switch/1
  [NegFlag] -> Switch/2
  Add/1 -> Switch/3
  Switch/1 -> Saturation Dynamic/2
  [UCell] -> MATLAB Function2/2(uCell)
  Constant22/1 -> MATLAB Function2/4(socBuffer)
  MATLAB Function2/1(enableOcv) -> [enableOcv]
  Constant30/1 -> MATLAB Function2/3(diffVMin)
  DCapacity/1 -> Switch6/1, Switch4/3
  Switch6/1 -> Switch5/3
  Logical Operator4/1 -> Switch6/2
  Divide16/1 -> MinMax1/1
  Constant25/1 -> MinMax1/2

== system Udan_SOC/SOC_Calculate/UdanSOCCalcn/SetSOHCalcFlag ==
  SocParam : Inport
  Trigger : TriggerPort  VariantControl=Variant
  Constant2 : Constant  Value=0  OutDataTypeStr=uint32
  Constant3 : Constant  Value=SOC_SOCResolution  OutDataTypeStr=uint16
  Constant31 : Constant  Value=SOC_NominalCap_AmS
  DchgPower1 : simulink/Sources/Enumerated Constant  OutDataTypeStr=Enum: ParameterM_EeepParaIndexType  Value=ParameterM_EeepParaIndexType.PARAMETERM_EEEP_SOH_Full_INDEX  SampleTime=inf
      settings: SourceProductName=Simulink
  DchgPower2 : simulink/Sources/Enumerated Constant  OutDataTypeStr=Enum: ParameterM_EeepParaIndexType  Value=ParameterM_EeepParaIndexType.PARAMETERM_EEEP_LEFTCAP_WOCALIB_H_INDEX  SampleTime=inf
      settings: SourceProductName=Simulink
  DchgPower4 : simulink/Sources/Enumerated Constant  OutDataTypeStr=Enum: ParameterM_EeepParaIndexType  Value=ParameterM_EeepParaIndexType.PARAMETERM_EEEP_LEFTCAP_WOCALIB_L_INDEX  SampleTime=inf
      settings: SourceProductName=Simulink
  Divide : Product  Inputs=*/  OutDataTypeStr=uint16
  Divide1 : Product  Inputs=*/  OutDataTypeStr=uint32
  S-Function1 : S-Function  FunctionName=sfn_NVMWrite  SFunctionDeploymentMode=off  EnableBusSupport=off
  Subsystem : Subsystem  mask(EeepWrite_uint32){}
      mask help: EeepWrite_uint32
  Terminator : Terminator
  wires:
  DchgPower1/1 -> S-Function1/1
  SocParam/1 -> Divide/1
  S-Function1/1 -> Terminator/1
  Divide/1 -> S-Function1/2
  DchgPower2/1 -> Subsystem/2(HighIndex)
  DchgPower4/1 -> Subsystem/3(LowIndex)
  Constant2/1 -> Subsystem/1(data)
  Constant3/1 -> Divide1/2
  Divide1/1 -> Divide/2
  Constant31/1 -> Divide1/1

== system Udan_SOC/SOC_Calculate/UdanSOCCalcn/SetSOHCalcFlagFullChg ==
  LastCap : Inport
  Trigger : TriggerPort  VariantControl=Variant
  Constant : Constant  OutDataTypeStr=boolean
  Constant2 : Constant  Value=SOC_SOCResolution  OutDataTypeStr=uint16
  Constant3 : Constant  Value=0  OutDataTypeStr=uint32
  Constant31 : Constant  Value=SOC_NominalCap_AmS
  Data Store Write : DataStoreWrite  DataStoreName=FullFnshFlag
  DchgPower1 : simulink/Sources/Enumerated Constant  OutDataTypeStr=Enum: ParameterM_EeepParaIndexType  Value=ParameterM_EeepParaIndexType.PARAMETERM_EEEP_SOH_Full_INDEX  SampleTime=inf
      settings: SourceProductName=Simulink
  DchgPower2 : simulink/Sources/Enumerated Constant  OutDataTypeStr=Enum: ParameterM_EeepParaIndexType  Value=ParameterM_EeepParaIndexType.PARAMETERM_EEEP_LEFTCAP_WOCALIB_H_INDEX  SampleTime=inf
      settings: SourceProductName=Simulink
  DchgPower4 : simulink/Sources/Enumerated Constant  OutDataTypeStr=Enum: ParameterM_EeepParaIndexType  Value=ParameterM_EeepParaIndexType.PARAMETERM_EEEP_LEFTCAP_WOCALIB_L_INDEX  SampleTime=inf
      settings: SourceProductName=Simulink
  Divide : Product  Inputs=*/  OutDataTypeStr=uint16
  Divide1 : Product  Inputs=*/  OutDataTypeStr=uint32
  S-Function1 : S-Function  FunctionName=sfn_NVMWrite  SFunctionDeploymentMode=off  EnableBusSupport=off
  Subsystem : Subsystem  mask(EeepWrite_uint32){}
      mask help: EeepWrite_uint32
  Terminator : Terminator
  wires:
  DchgPower1/1 -> S-Function1/1
  Constant31/1 -> Divide1/1
  Divide1/1 -> Divide/2
  Constant2/1 -> Divide1/2
  S-Function1/1 -> Terminator/1
  Divide/1 -> S-Function1/2
  LastCap/1 -> Divide/1
  Constant/1 -> Data Store Write/1
  DchgPower2/1 -> Subsystem/2(HighIndex)
  DchgPower4/1 -> Subsystem/3(LowIndex)
  Constant3/1 -> Subsystem/1(data)
